simulink model "Product"  (Simulink 8.0)
settings: Solver=ode45  StartTime=0.0  StopTime=10.0  RelTol=1e-3
settings Model: Creator=Faradars  LastModifiedBy=Faradars

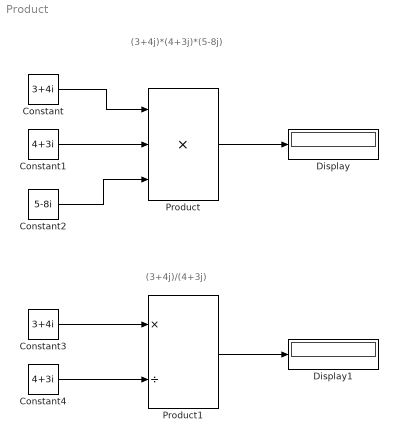
== system Product ==
  note: (3+4j)/(4+3j)
  note: (3+4j)*(4+3j)*(5-8j)
  Constant : Constant  Value=3+4i
  Constant1 : Constant  Value=4+3i
  Constant2 : Constant  Value=5-8i
  Constant3 : Constant  Value=3+4i
  Constant4 : Constant  Value=4+3i
  Display : Display
  Display1 : Display
  Product : Product  Inputs=3  RndMeth=Zero
  Product1 : Product  Inputs=*/  RndMeth=Zero
  wires:
  Constant/1 -> Product/1
  Constant1/1 -> Product/2
  Constant2/1 -> Product/3
  Product/1 -> Display/1
  Constant3/1 -> Product1/1
  Constant4/1 -> Product1/2
  Product1/1 -> Display1/1
